simulink model "gm_sampleModel1727_3_sub"  (R2023a)
settings: Solver=VariableStepAuto  StartTime=0.0  StopTime=10.0  RelTol=1e-3
libraries: simulink x4, hdlsllib x1
settings Model: Creator=user1  LastModifiedBy=user1
settings OptimizationCC: BlockReduction=off  ConditionallyExecuteInputs=off
settings DebuggingCC: InheritedTsInSrcMsg=none

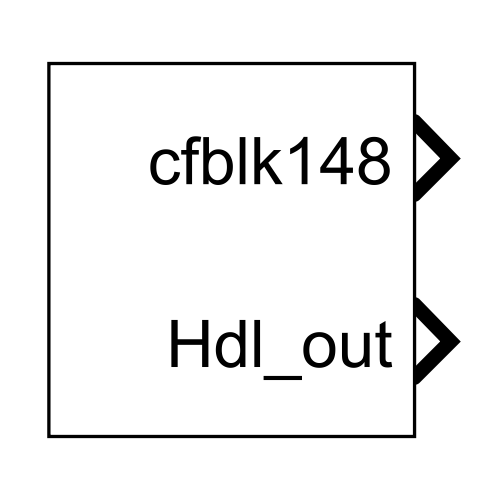
[thumbnail: Simulink's stored preview of the top-level diagram]
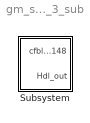
== system gm_sampleModel1727_3_sub ==
  Subsystem : Subsystem

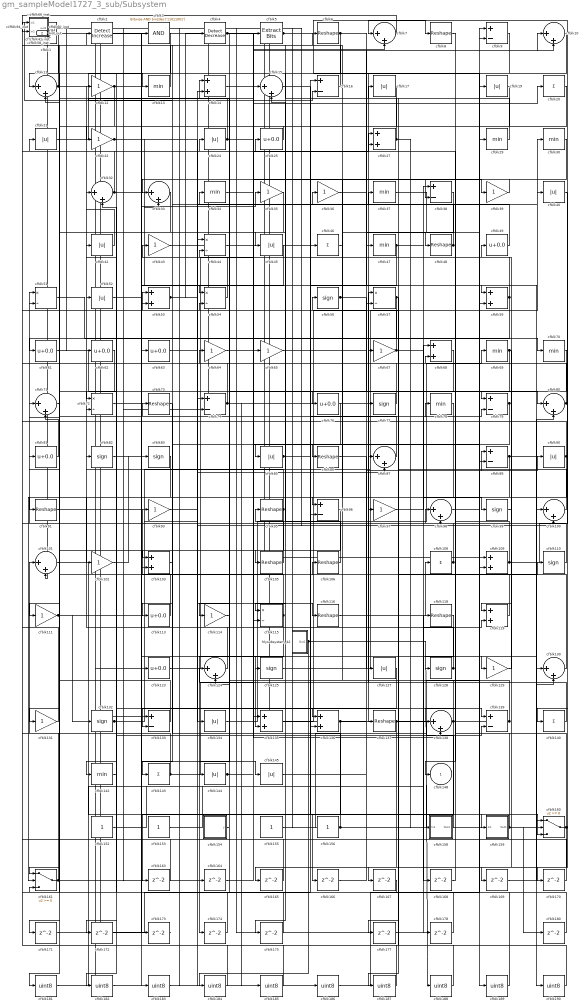
== system gm_sampleModel1727_3_sub/Subsystem ==
  Mysubsystem_42 : Subsystem
  cfblk1 : hdlsllib/Logic and Bit Operations/Interval Test  IntervalClosedRight=on  uplimit=0.5  IntervalClosedLeft=on  lowlimit=-0.5  OutDataTypeStr=uint8
  cfblk{7,10..11,15,32..33,71,80,87,98,100..101,124,130,138} (15 alike) : Sum  Inputs=|++  OutDataTypeStr=uint8
  cfblk{12,22,35..36,39,43,64..65,67,93,97,102,111,114,129,131} (16 alike) : Gain  OutDataTypeStr=uint8
  cfblk{14,27,53,59,68,103,109,119,135..136} (10 alike) : Sum  OutDataTypeStr=uint8
  cfblk{6,8,48,73,86,91,95,105..106,116,118,137} (12 alike) : Reshape
  cfblk{20,46,108,140,143} (5 alike) : Sum  Inputs=+  OutDataTypeStr=uint8
  cfblk{56,77,82..83,99,110,125,128,132} (9 alike) : Signum
  cfblk{25,49,61..63,76,81,113,123} (9 alike) : Bias  Bias=0.0  SaturateOnIntegerOverflow=off
  cfblk{44,51,54,57,72,115} (6 alike) : Product  Inputs=*/  OutDataTypeStr=uint8  RndMeth=Zero  SaturateOnIntegerOverflow=on
  cfblk117_inst : Subsystem
  cfblk120_inst : Subsystem
  cfblk121_inst : Subsystem
  cfblk{17,19,21,24,40,42,45,52,85,90,127,134,144..145} (14 alike) : Abs  OutDataTypeStr=uint8  SaturateOnIntegerOverflow=off
  cfblk{13,29..30,34,37,47,69..70,78,142} (10 alike) : MinMax  OutDataTypeStr=uint8
  cfblk{9,16,38,74,79,89,96,133,139} (9 alike) : Sum  Inputs=+-  OutDataTypeStr=uint8
  cfblk146_inst : Subsystem
  cfblk{152..153,155..156} (4 alike) : Constant  OutDataTypeStr=uint8  SampleTime=-1
  cfblk154 : Subsystem  mask(Counter Free-Running){NumBits=double(16), tsamp=double(-1)}
      mask prompts: NumBits "Simulink:masks:NumberOfBits_MP"; tsamp "Simulink:masks:SampleTime_MP"
      mask help: Simulink:masks:CounterFreeRunning_MD
  cfblk158 : Subsystem
  cfblk159 : Subsystem
  cfblk160 : Switch  OutDataTypeStr=uint8  SaturateOnIntegerOverflow=off  InputSameDT=off
  cfblk161 : Switch  OutDataTypeStr=uint8  SaturateOnIntegerOverflow=off  InputSameDT=off
  cfblk{163..175,177..178,180} (16 alike) : Delay  SampleTime=1
  cfblk{181..190} (10 alike) : DataTypeConversion  OutDataTypeStr=uint8  SaturateOnIntegerOverflow=off  RndMeth=Floor
  cfblk18_inst : Subsystem
  cfblk2 : simulink/Logic and Bit Operations/Detect Increase  vinit=0.0  OutDataTypeStr=uint8
      settings: LibrarySourceBlock=|
      | hdlsllib/Logic and Bit
      | Operations/Detect
      | Increase
  cfblk23_inst : Subsystem
  cfblk28_inst : Subsystem
  cfblk3 : simulink/Logic and Bit Operations/Bitwise Operator  logicop=AND  UseBitMask=on  BitMask=bin2dec('11011001')  BitMaskRealWorld=Stored Integer
      settings: LibrarySourceBlock=|
      | hdlsllib/Logic and Bit
      | Operations/Bitwise
      | Operator
  cfblk4 : simulink/Logic and Bit Operations/Detect Decrease  vinit=0.0  OutDataTypeStr=uint8
      settings: LibrarySourceBlock=|
      | hdlsllib/Logic and Bit
      | Operations/Detect
      | Decrease
  cfblk41_inst : Subsystem
  cfblk5 : simulink/Logic and Bit Operations/Extract Bits  bitsToExtract=Upper half  numBits=8  bitIdxRange=[0 7]  outScalingMode=Preserve fixed-point scaling
      settings: LibrarySourceBlock=|
      | hdlsllib/Logic and Bit
      | Operations/Extract Bits
  cfblk58_inst : Subsystem
  cfblk60_inst : Subsystem
  cfblk66_inst : Subsystem
  cfblk94_inst : Subsystem
  cfblk148 : Outport  OutDataTypeStr=uint8  SampleTime=1  VectorParamsAs1DForOutWhenUnconnected=off
  Hdl_out : Outport  Port=2  OutDataTypeStr=uint8  SampleTime=1
  wires:
  Mysubsystem_42/1(Out1) -> cfblk188/1, cfblk184/1, cfblk133/2
  cfblk1/1 -> cfblk11/1
  cfblk10/1 -> cfblk137/1
  cfblk100/1 -> cfblk56/1
  cfblk101/1 -> cfblk160/3
  cfblk102/1 -> cfblk83/1
  cfblk103/1 -> cfblk60_inst/1(in1)
  cfblk105/1 -> cfblk95/1
  cfblk106/1 -> cfblk25/1
  cfblk108/1 -> cfblk94_inst/1(in1), cfblk57/1
  cfblk109/1 -> cfblk7/1, cfblk44/2
  cfblk11/1 -> cfblk28_inst/2(in2), cfblk16/2, cfblk13/1
  cfblk110/1 -> cfblk51/1
  cfblk111/1 -> cfblk132/1, cfblk30/1
  cfblk113/1 -> cfblk93/1
  cfblk114/1 -> cfblk14/1
  cfblk115/1 -> cfblk94_inst/2(in2), cfblk135/2, cfblk174/1
  cfblk116/1 -> cfblk108/1
  cfblk117_inst/1(out1) -> cfblk183/1
  cfblk118/1 -> cfblk128/1
  cfblk119/1 -> cfblk27/1
  cfblk12/1 -> cfblk91/1, cfblk145/1
  cfblk120_inst/1(out1) -> cfblk109/1
  cfblk121_inst/1(out1) -> cfblk160/2, cfblk178/1
  cfblk123/1 -> cfblk15/1
  cfblk124/1 -> cfblk12/1
  cfblk125/1 -> cfblk89/1
  cfblk127/1 -> cfblk142/1
  cfblk128/1 -> cfblk73/1, cfblk24/1
  cfblk129/1 -> cfblk49/1
  cfblk13/1 -> cfblk120_inst/2(in2)
  cfblk130/1 -> cfblk68/2
  cfblk131/1 -> cfblk121_inst/1(in1)
  cfblk132/1 -> cfblk63/1, cfblk14/2
  cfblk133/1 -> cfblk81/1
  cfblk134/1 -> cfblk69/1
  cfblk135/1 -> cfblk47/1
  cfblk136/1 -> cfblk90/1, cfblk163/1
  cfblk137/1 -> cfblk139/2, cfblk167/1
  cfblk138/1 -> cfblk36/1, cfblk166/1
  cfblk139/1 -> cfblk53/1, cfblk124/1, Hdl_out/1
  cfblk14/1 -> cfblk70/1
  cfblk140/1 -> cfblk87/1
  cfblk142/1 -> cfblk32/2
  cfblk143/1 -> cfblk5/1, cfblk101/1
  cfblk144/1 -> cfblk135/1, cfblk64/1
  cfblk145/1 -> cfblk57/2
  cfblk146_inst/1(out1) -> cfblk74/2, cfblk46/1
  cfblk15/1 -> cfblk160/1
  cfblk152/1 -> cfblk65/1
  cfblk153/1 -> cfblk118/1
  cfblk154/1(y) -> cfblk34/1
  cfblk155/1 -> cfblk9/1
  cfblk156/1 -> cfblk19/1, cfblk103/2
  cfblk158/1(Out1) -> cfblk52/1
  cfblk159/1(Out1) -> cfblk80/2, cfblk97/1, cfblk180/1
  cfblk16/1 -> cfblk66_inst/2(in2)
  cfblk160/1 -> cfblk21/1, cfblk165/1
  cfblk161/1 -> cfblk146_inst/1(in1), cfblk35/1
  cfblk163/1 -> cfblk66_inst/1(in1)
  cfblk164/1 -> cfblk27/2
  cfblk165/1 -> cfblk11/2
  cfblk166/1 -> cfblk79/2
  cfblk167/1 -> cfblk161/3
  cfblk168/1 -> cfblk98/1
  cfblk169/1 -> cfblk100/1
  cfblk17/1 -> cfblk175/1
  cfblk170/1 -> cfblk71/1
  cfblk171/1 -> cfblk44/1
  cfblk172/1 -> cfblk16/1
  cfblk173/1 -> cfblk1/1
  cfblk174/1 -> cfblk72/2
  cfblk175/1 -> cfblk51/2
  cfblk177/1 -> cfblk119/2
  cfblk178/1 -> cfblk54/2
  cfblk18_inst/1(out1) -> cfblk186/1
  cfblk180/1 -> cfblk74/1
  cfblk181/1 -> cfblk3/1
  cfblk182/1 -> cfblk110/1
  cfblk183/1 -> cfblk106/1
  cfblk184/1 -> cfblk117_inst/1(in1)
  cfblk185/1 -> cfblk117_inst/2(in2)
  cfblk186/1 -> cfblk9/2
  cfblk187/1 -> cfblk18_inst/1(in1)
  cfblk188/1 -> cfblk18_inst/2(in2)
  cfblk189/1 -> cfblk60_inst/2(in2)
  cfblk19/1 -> cfblk45/1
  cfblk190/1 -> cfblk37/1
  cfblk2/1 -> cfblk125/1
  cfblk20/1 -> cfblk172/1
  cfblk21/1 -> cfblk7/2
  cfblk22/1 -> cfblk87/2, cfblk33/2
  cfblk23_inst/1(out1) -> cfblk101/2
  cfblk24/1 -> cfblk59/1, cfblk23_inst/1(in1), cfblk138/2
  cfblk25/1 -> cfblk22/1
  cfblk27/1 -> cfblk146_inst/2(in2), cfblk158/1(In1)
  cfblk28_inst/1(out1) -> cfblk123/1
  cfblk29/1 -> cfblk2/1
  cfblk3/1 -> cfblk182/1
  cfblk30/1 -> cfblk96/1
  cfblk32/1 -> cfblk130/1, cfblk121_inst/2(in2)
  cfblk33/1 -> cfblk61/1
  cfblk34/1 -> cfblk89/2
  cfblk35/1 -> cfblk72/1
  cfblk36/1 -> cfblk48/1
  cfblk37/1 -> cfblk189/1
  cfblk38/1 -> cfblk76/1
  cfblk39/1 -> cfblk33/1
  cfblk4/1 -> cfblk124/2, cfblk39/1
  cfblk40/1 -> cfblk170/1
  cfblk41_inst/1(out1) -> cfblk77/1
  cfblk42/1 -> cfblk32/1
  cfblk43/1 -> cfblk98/2
  cfblk44/1 -> cfblk10/1
  cfblk45/1 -> cfblk53/2
  cfblk46/1 -> cfblk86/1
  cfblk47/1 -> cfblk99/1, cfblk96/2, cfblk40/1
  cfblk48/1 -> cfblk23_inst/2(in2), cfblk120_inst/1(in1)
  cfblk49/1 -> cfblk17/1
  cfblk5/1 -> cfblk8/1, cfblk109/2
  cfblk51/1 -> cfblk67/1
  cfblk52/1 -> cfblk54/1
  cfblk53/1 -> cfblk116/1, cfblk4/1
  cfblk54/1 -> cfblk43/1
  cfblk56/1 -> cfblk80/1, cfblk79/1
  cfblk57/1 -> cfblk177/1, cfblk114/1
  cfblk58_inst/1(out1) -> cfblk164/1
  cfblk59/1 -> cfblk15/2, cfblk131/1
  cfblk6/1 -> cfblk59/2, cfblk38/2, cfblk111/1
  cfblk60_inst/1(out1) -> cfblk133/1
  cfblk61/1 -> cfblk168/1
  cfblk62/1 -> cfblk181/1
  cfblk63/1 -> cfblk38/1
  cfblk64/1 -> cfblk20/1
  cfblk65/1 -> cfblk10/2
  cfblk66_inst/1(out1) -> cfblk100/2
  cfblk67/1 -> cfblk28_inst/1(in1), cfblk129/1
  cfblk68/1 -> cfblk144/1
  cfblk69/1 -> cfblk119/1, cfblk148/1
  cfblk7/1 -> cfblk58_inst/2(in2)
  cfblk70/1 -> cfblk187/1
  cfblk71/1 -> cfblk161/1
  cfblk72/1 -> cfblk136/1
  cfblk73/1 -> cfblk103/1
  cfblk74/1 -> cfblk42/1, cfblk185/1, cfblk159/1(In1)
  cfblk76/1 -> cfblk115/1
  cfblk77/1 -> cfblk6/1
  cfblk78/1 -> cfblk102/1
  cfblk79/1 -> cfblk85/1, cfblk113/1
  cfblk8/1 -> cfblk138/1
  cfblk80/1 -> cfblk41_inst/1(in1), cfblk140/1
  cfblk81/1 -> cfblk71/2
  cfblk82/1 -> cfblk173/1
  cfblk83/1 -> cfblk161/2
  cfblk85/1 -> cfblk139/1, cfblk78/1
  cfblk86/1 -> cfblk127/1
  cfblk87/1 -> cfblk58_inst/1(in1)
  cfblk89/1 -> cfblk190/1, cfblk136/2
  cfblk9/1 -> cfblk105/1
  cfblk90/1 -> cfblk41_inst/2(in2), cfblk143/1
  cfblk91/1 -> cfblk130/2
  cfblk93/1 -> cfblk134/1
  cfblk94_inst/1(out1) -> cfblk62/1
  cfblk95/1 -> cfblk82/1, cfblk115/2
  cfblk96/1 -> cfblk171/1
  cfblk97/1 -> cfblk68/1
  cfblk98/1 -> cfblk29/1
  cfblk99/1 -> cfblk169/1

== system gm_sampleModel1727_3_sub/Subsystem/Mysubsystem_42 ==
  cfblk157 : Subsystem  mask(Counter Limited){uplimit=double(7), tsamp=double(-1)}
      mask prompts: uplimit "Simulink:masks:UpperLimit_MP"; tsamp "Simulink:masks:SampleTime_MP"
      mask help: Simulink:masks:CounterLimited_MD
      mask init:
      | nbits = double(8);
      | tsamp = double(-1);
      | uplimit = double(7);
  cfblk84 : Sum  Inputs=+
  Out1 : Outport  SampleTime=1
  wires:
  cfblk157/1(y) -> cfblk84/1
  cfblk84/1 -> Out1/1

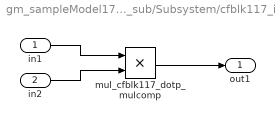
== system gm_sampleModel1727_3_sub/Subsystem/cfblk117_inst ==
  in1 : Inport  OutDataTypeStr=uint8  SampleTime=1
  in2 : Inport  Port=2  OutDataTypeStr=uint8  SampleTime=1
  mul_cfblk117_dotp_mulcomp : Product  Inputs=**  OutDataTypeStr=uint8  SampleTime=1
  out1 : Outport  OutDataTypeStr=uint8  SampleTime=1
  wires:
  in1/1 -> mul_cfblk117_dotp_mulcomp/1
  in2/1 -> mul_cfblk117_dotp_mulcomp/2
  mul_cfblk117_dotp_mulcomp/1 -> out1/1

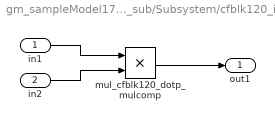
== system gm_sampleModel1727_3_sub/Subsystem/cfblk120_inst ==
  in1 : Inport  OutDataTypeStr=uint8  SampleTime=1
  in2 : Inport  Port=2  OutDataTypeStr=uint8  SampleTime=1
  mul_cfblk120_dotp_mulcomp : Product  Inputs=**  OutDataTypeStr=uint8  SampleTime=1
  out1 : Outport  OutDataTypeStr=uint8  SampleTime=1
  wires:
  in1/1 -> mul_cfblk120_dotp_mulcomp/1
  in2/1 -> mul_cfblk120_dotp_mulcomp/2
  mul_cfblk120_dotp_mulcomp/1 -> out1/1

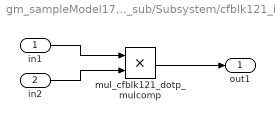
== system gm_sampleModel1727_3_sub/Subsystem/cfblk121_inst ==
  in1 : Inport  OutDataTypeStr=uint8  SampleTime=1
  in2 : Inport  Port=2  OutDataTypeStr=uint8  SampleTime=1
  mul_cfblk121_dotp_mulcomp : Product  Inputs=**  OutDataTypeStr=uint8  SampleTime=1
  out1 : Outport  OutDataTypeStr=uint8  SampleTime=1
  wires:
  in1/1 -> mul_cfblk121_dotp_mulcomp/1
  in2/1 -> mul_cfblk121_dotp_mulcomp/2
  mul_cfblk121_dotp_mulcomp/1 -> out1/1

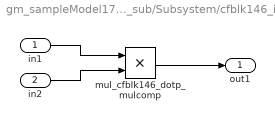
== system gm_sampleModel1727_3_sub/Subsystem/cfblk146_inst ==
  in1 : Inport  OutDataTypeStr=uint8  SampleTime=1
  in2 : Inport  Port=2  OutDataTypeStr=uint8  SampleTime=1
  mul_cfblk146_dotp_mulcomp : Product  Inputs=**  OutDataTypeStr=uint8  SampleTime=1
  out1 : Outport  OutDataTypeStr=uint8  SampleTime=1
  wires:
  in1/1 -> mul_cfblk146_dotp_mulcomp/1
  in2/1 -> mul_cfblk146_dotp_mulcomp/2
  mul_cfblk146_dotp_mulcomp/1 -> out1/1

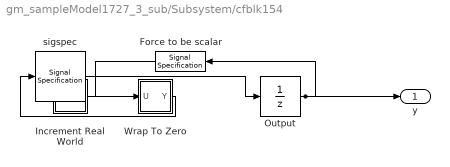
== system gm_sampleModel1727_3_sub/Subsystem/cfblk154 ==
  Force to be scalar : SignalSpecification  DisableCoverage=on  Dimensions=1
  Increment Real World : Subsystem  mask(Real World Value Increment){}
      mask help: Simulink:masks:RealWorldValueIncrement_MD
      mask Display: disp('V++')
  Output : UnitDelay  InitialCondition=0.0  SampleTime=tsamp  HasFrameUpgradeWarning=on
  Wrap To Zero : Subsystem  mask(Wrap To Zero){Threshold=double(65535)}
      mask prompts: Threshold "Simulink:masks:Threshold_MP"
      mask help: Simulink:masks:WrapToZero_MD
  sigspec : SignalSpecification  OutDataTypeStr=uint16  Dimensions=1
  y : Outport  SampleTime=1
  wires:
  Force to be scalar/1 -> Increment Real World/1(u)
  Increment Real World/1(y) -> Wrap To Zero/1(U)
  Output/1 -> Force to be scalar/1, y/1
  Wrap To Zero/1(Y) -> sigspec/1
  sigspec/1 -> Output/1

== system gm_sampleModel1727_3_sub/Subsystem/cfblk158 ==
  In1 : Inport  OutDataTypeStr=uint8  PortDimensions=1  SampleTime=1
  Out1 : Outport  SampleTime=1
  wires:
  In1/1 -> Out1/1

== system gm_sampleModel1727_3_sub/Subsystem/cfblk159 ==
  In1 : Inport  OutDataTypeStr=uint8  PortDimensions=1  SampleTime=1
  Out1 : Outport  SampleTime=1
  wires:
  In1/1 -> Out1/1

== system gm_sampleModel1727_3_sub/Subsystem/cfblk18_inst ==
  in1 : Inport  OutDataTypeStr=uint8  SampleTime=1
  in2 : Inport  Port=2  OutDataTypeStr=uint8  SampleTime=1
  mul_cfblk18_dotp_mulcomp : Product  Inputs=**  OutDataTypeStr=uint8  SampleTime=1
  out1 : Outport  OutDataTypeStr=uint8  SampleTime=1
  wires:
  in1/1 -> mul_cfblk18_dotp_mulcomp/1
  in2/1 -> mul_cfblk18_dotp_mulcomp/2
  mul_cfblk18_dotp_mulcomp/1 -> out1/1

== system gm_sampleModel1727_3_sub/Subsystem/cfblk23_inst ==
  in1 : Inport  OutDataTypeStr=uint8  SampleTime=1
  in2 : Inport  Port=2  OutDataTypeStr=uint8  SampleTime=1
  mul_cfblk23_dotp_mulcomp : Product  Inputs=**  OutDataTypeStr=uint8  SampleTime=1
  out1 : Outport  OutDataTypeStr=uint8  SampleTime=1
  wires:
  in1/1 -> mul_cfblk23_dotp_mulcomp/1
  in2/1 -> mul_cfblk23_dotp_mulcomp/2
  mul_cfblk23_dotp_mulcomp/1 -> out1/1

== system gm_sampleModel1727_3_sub/Subsystem/cfblk28_inst ==
  in1 : Inport  OutDataTypeStr=uint8  SampleTime=1
  in2 : Inport  Port=2  OutDataTypeStr=uint8  SampleTime=1
  mul_cfblk28_dotp_mulcomp : Product  Inputs=**  OutDataTypeStr=uint8  SampleTime=1
  out1 : Outport  OutDataTypeStr=uint8  SampleTime=1
  wires:
  in1/1 -> mul_cfblk28_dotp_mulcomp/1
  in2/1 -> mul_cfblk28_dotp_mulcomp/2
  mul_cfblk28_dotp_mulcomp/1 -> out1/1

== system gm_sampleModel1727_3_sub/Subsystem/cfblk41_inst ==
  in1 : Inport  OutDataTypeStr=uint8  SampleTime=1
  in2 : Inport  Port=2  OutDataTypeStr=uint8  SampleTime=1
  mul_cfblk41_dotp_mulcomp : Product  Inputs=**  OutDataTypeStr=uint8  SampleTime=1
  out1 : Outport  OutDataTypeStr=uint8  SampleTime=1
  wires:
  in1/1 -> mul_cfblk41_dotp_mulcomp/1
  in2/1 -> mul_cfblk41_dotp_mulcomp/2
  mul_cfblk41_dotp_mulcomp/1 -> out1/1

== system gm_sampleModel1727_3_sub/Subsystem/cfblk58_inst ==
  in1 : Inport  OutDataTypeStr=uint8  SampleTime=1
  in2 : Inport  Port=2  OutDataTypeStr=uint8  SampleTime=1
  mul_cfblk58_dotp_mulcomp : Product  Inputs=**  OutDataTypeStr=uint8  SampleTime=1
  out1 : Outport  OutDataTypeStr=uint8  SampleTime=1
  wires:
  in1/1 -> mul_cfblk58_dotp_mulcomp/1
  in2/1 -> mul_cfblk58_dotp_mulcomp/2
  mul_cfblk58_dotp_mulcomp/1 -> out1/1

== system gm_sampleModel1727_3_sub/Subsystem/cfblk60_inst ==
  in1 : Inport  OutDataTypeStr=uint8  SampleTime=1
  in2 : Inport  Port=2  OutDataTypeStr=uint8  SampleTime=1
  mul_cfblk60_dotp_mulcomp : Product  Inputs=**  OutDataTypeStr=uint8  SampleTime=1
  out1 : Outport  OutDataTypeStr=uint8  SampleTime=1
  wires:
  in1/1 -> mul_cfblk60_dotp_mulcomp/1
  in2/1 -> mul_cfblk60_dotp_mulcomp/2
  mul_cfblk60_dotp_mulcomp/1 -> out1/1

== system gm_sampleModel1727_3_sub/Subsystem/cfblk66_inst ==
  in1 : Inport  OutDataTypeStr=uint8  SampleTime=1
  in2 : Inport  Port=2  OutDataTypeStr=uint8  SampleTime=1
  mul_cfblk66_dotp_mulcomp : Product  Inputs=**  OutDataTypeStr=uint8  SampleTime=1
  out1 : Outport  OutDataTypeStr=uint8  SampleTime=1
  wires:
  in1/1 -> mul_cfblk66_dotp_mulcomp/1
  in2/1 -> mul_cfblk66_dotp_mulcomp/2
  mul_cfblk66_dotp_mulcomp/1 -> out1/1

== system gm_sampleModel1727_3_sub/Subsystem/cfblk94_inst ==
  in1 : Inport  OutDataTypeStr=uint8  SampleTime=1
  in2 : Inport  Port=2  OutDataTypeStr=uint8  SampleTime=1
  mul_cfblk94_dotp_mulcomp : Product  Inputs=**  OutDataTypeStr=uint8  SampleTime=1
  out1 : Outport  OutDataTypeStr=uint8  SampleTime=1
  wires:
  in1/1 -> mul_cfblk94_dotp_mulcomp/1
  in2/1 -> mul_cfblk94_dotp_mulcomp/2
  mul_cfblk94_dotp_mulcomp/1 -> out1/1

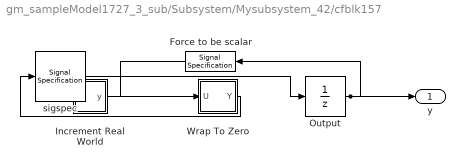
== system gm_sampleModel1727_3_sub/Subsystem/Mysubsystem_42/cfblk157 ==
  Force to be scalar : SignalSpecification  DisableCoverage=on  Dimensions=1
  Increment Real World : Subsystem  mask(Real World Value Increment){}
      mask help: Simulink:masks:RealWorldValueIncrement_MD
      mask Display: disp('V++')
  Output : UnitDelay  InitialCondition=0.0  SampleTime=tsamp  HasFrameUpgradeWarning=on
  Wrap To Zero : Subsystem  mask(Wrap To Zero){Threshold=double(7)}
      mask prompts: Threshold "Simulink:masks:Threshold_MP"
      mask help: Simulink:masks:WrapToZero_MD
  sigspec : SignalSpecification  OutDataTypeStr=uint8  Dimensions=1
  y : Outport  SampleTime=1
  wires:
  Force to be scalar/1 -> Increment Real World/1(u)
  Increment Real World/1(y) -> Wrap To Zero/1(U)
  Output/1 -> Force to be scalar/1, y/1
  Wrap To Zero/1(Y) -> sigspec/1
  sigspec/1 -> Output/1

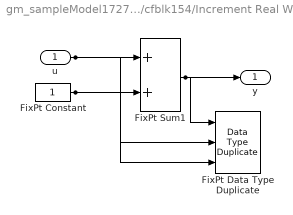
== system gm_sampleModel1727_3_sub/Subsystem/cfblk154/Increment Real World ==
  u : Inport  OutDataTypeStr=uint16  SampleTime=1
  FixPt Constant : Constant  DisableCoverage=on  OutDataTypeStr=Inherit: Inherit via back propagation  SampleTime=-1
  FixPt Data Type Duplicate : DataTypeDuplicate  DisableCoverage=on  NumInputPorts=3
  FixPt Sum1 : Sum  InputSameDT=on  OutDataTypeStr=Inherit: Inherit via back propagation  LockScale=on
  y : Outport  SampleTime=1
  wires:
  u/1 -> FixPt Sum1/1, FixPt Data Type Duplicate/2
  FixPt Constant/1 -> FixPt Sum1/2, FixPt Data Type Duplicate/3
  FixPt Sum1/1 -> FixPt Data Type Duplicate/1, y/1

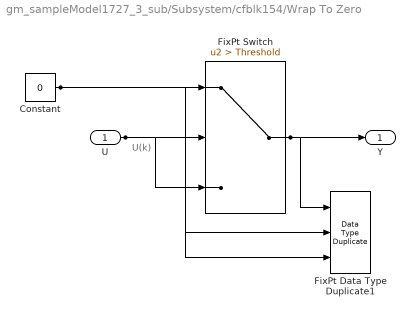
== system gm_sampleModel1727_3_sub/Subsystem/cfblk154/Wrap To Zero ==
  note: U(k)
  U : Inport  OutDataTypeStr=uint16  SampleTime=1
  Constant : Constant  DisableCoverage=on  Value=0  OutDataTypeStr=Inherit: Inherit via back propagation  SampleTime=-1
  FixPt Data Type Duplicate1 : DataTypeDuplicate  DisableCoverage=on  NumInputPorts=3
  FixPt Switch : Switch  Criteria=u2 > Threshold  Threshold=Threshold  OutDataTypeStr=Inherit: Inherit via back propagation  ZeroCross=off  SaturateOnIntegerOverflow=off  InputSameDT=off
  Y : Outport  SampleTime=1
  wires:
  U/1 -> FixPt Switch/3, FixPt Switch/2, FixPt Data Type Duplicate1/2
  Constant/1 -> FixPt Switch/1, FixPt Data Type Duplicate1/3
  FixPt Switch/1 -> FixPt Data Type Duplicate1/1, Y/1

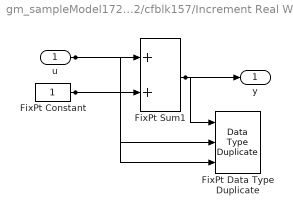
== system gm_sampleModel1727_3_sub/Subsystem/Mysubsystem_42/cfblk157/Increment Real World ==
  u : Inport  OutDataTypeStr=uint8  SampleTime=1
  FixPt Constant : Constant  DisableCoverage=on  OutDataTypeStr=Inherit: Inherit via back propagation  SampleTime=-1
  FixPt Data Type Duplicate : DataTypeDuplicate  DisableCoverage=on  NumInputPorts=3
  FixPt Sum1 : Sum  InputSameDT=on  OutDataTypeStr=Inherit: Inherit via back propagation  LockScale=on
  y : Outport  SampleTime=1
  wires:
  u/1 -> FixPt Sum1/1, FixPt Data Type Duplicate/2
  FixPt Constant/1 -> FixPt Sum1/2, FixPt Data Type Duplicate/3
  FixPt Sum1/1 -> FixPt Data Type Duplicate/1, y/1

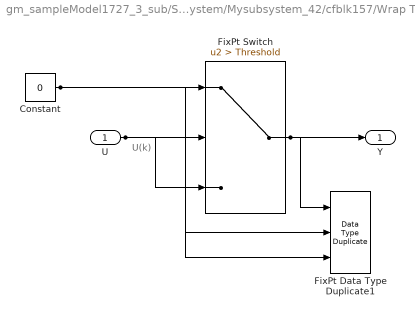
== system gm_sampleModel1727_3_sub/Subsystem/Mysubsystem_42/cfblk157/Wrap To Zero ==
  note: U(k)
  U : Inport  OutDataTypeStr=uint8  SampleTime=1
  Constant : Constant  DisableCoverage=on  Value=0  OutDataTypeStr=Inherit: Inherit via back propagation  SampleTime=-1
  FixPt Data Type Duplicate1 : DataTypeDuplicate  DisableCoverage=on  NumInputPorts=3
  FixPt Switch : Switch  Criteria=u2 > Threshold  Threshold=Threshold  OutDataTypeStr=Inherit: Inherit via back propagation  ZeroCross=off  SaturateOnIntegerOverflow=off  InputSameDT=off
  Y : Outport  SampleTime=1
  wires:
  U/1 -> FixPt Switch/3, FixPt Switch/2, FixPt Data Type Duplicate1/2
  Constant/1 -> FixPt Switch/1, FixPt Data Type Duplicate1/3
  FixPt Switch/1 -> FixPt Data Type Duplicate1/1, Y/1
